simulink model "testbench_str1"  (R2015a)
settings: Solver=ode3  StartTime=0.0  StopTime=50  RelTol=1e-3
libraries: legoev3lib x2
settings Model: SimulationMode=external  ExtModeTrigDuration=2  Creator=USER  LastModifiedBy=USER
settings SolverCC: PositivePriorityOrder=on
settings OptimizationCC: OptimizeModelRefInitCode=on  LifeSpan=Inf  MaxStackSize=64
settings DebuggingCC: UnderspecifiedInitializationDetection=Classic  MergeDetectMultiDrivingBlocksExec=none  ParameterTunabilityLossMsg=error
settings HardwareCC: ProdLargestAtomicInteger=Long  ProdLargestAtomicFloat=Float  ProdEndianess=LittleEndian  ProdHWDeviceType=ARM Compatible->ARM 9
settings RTWCC: SystemTargetFile=realtime.tlc  TLCOptions="-aInlineSetEventsForThisBaseRateFcn=TLC_FALSE  -aRateBasedStepFcn=0"  GenerateMakefile=off  TemplateMakefile=realtime.tmf  Description=Run on Target Hardware  RTWVerbose=off  IncludeHyperlinkInReport=on
settings CodeAppCC: ForceParamTrailComments=on  OperatorAnnotations=on  MATLABSourceComments=on
settings ERTTargetCC: CombineOutputUpdateFcns=off  ERTSrcFileBannerTemplate=realtime_code_template.cgt  ERTHdrFileBannerTemplate=realtime_code_template.cgt  ERTDataSrcFileTemplate=realtime_code_template.cgt  ERTDataHdrFileTemplate=realtime_code_template.cgt  ERTCustomFileTemplate=realtime_file_process.tlc

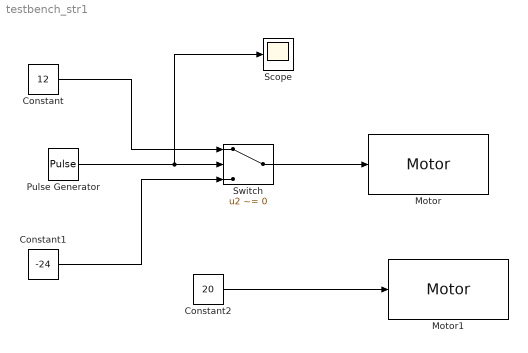
== system testbench_str1 ==
  Constant : Constant  Value=12
  Constant1 : Constant  Value=-24
  Constant2 : Constant  Value=20
  Motor : legoev3lib/Motor  sportNumber=B  sstopAction=Brake
  Motor1 : legoev3lib/Motor  sportNumber=A  sstopAction=Brake
  Pulse Generator : DiscretePulseGenerator  PulseType=Time based  PulseWidth=50
  Scope : Scope
      settings: TimeRange=0.126076464172133  YMin=0.95  YMax=1.05
  Switch : Switch  Criteria=u2 ~= 0
  wires:
  Switch/1 -> Motor/1
  Constant/1 -> Switch/1
  Constant1/1 -> Switch/3
  Pulse Generator/1 -> Scope/1, Switch/2
  Constant2/1 -> Motor1/1
